simulink model "ClimateControlSystem_Standalone"  (R2026a)
settings: Solver=FixedStepAuto  StopTime=300  FixedStep=0.001  MaxStep=1e-4  RelTol=1e-4  AbsTol=1e-4  EnableMultiTasking=on
PreLoadFcn:
  | % NXP_MBDT_S32K3 callback: DO NOT REMOVE
  | mbd_s32k3.common.nxp.model_callbacks.preLoadFcn();
PostLoadFcn:
  | % NXP_MBDT_S32K3 callback: DO NOT REMOVE
  | mbd_s32k3.common.nxp.model_callbacks.postLoadFcn();
InitFcn:
  | % NXP_MBDT_S32K3 callback: DO NOT REMOVE
  | mbd_s32k3.common.nxp.model_callbacks.initFcn();
undefined symbols (not defined in the file or in its folder): DiscIntNeverNeededParam
libraries: mbd_s32k3_io_library x12, mbd_s32k3_isr_library x2, mbd_s32k3_utility_library x1
settings Model: DataDictionary=ClimateControlSystem_Standalone.sldd  PacingRate=1.100000  ExtModeTrigMode=oneshot  ExtModeArmWhenConnect=off  Creator=The MathWorks, Inc.  LastModifiedBy=nxa06644
settings SolverCC: MinimalZcImpactIntegration=on
settings DataIOCC: SignalLoggingName=sigsOut
settings OptimizationCC: InitFltsAndDblsToZero=on  EfficientMapNaN2IntZero=off
settings DebuggingCC: AlgebraicLoopMsg=error  SaveWithParameterizedLinksMsg=none  MultiTaskDSMMsg=warning  MultiTaskCondExecSysMsg=none  SubsystemReferenceDiagnosticForUnitTest=warning
settings HardwareCC: ProdLargestAtomicInteger=Long  ProdLargestAtomicFloat=Double  ProdHWDeviceType=ARM Compatible->ARM Cortex
settings RTWCC: SystemTargetFile=ert.tlc  HardwareBoard=NXP S32K3xx  TLCOptions=-aInlineSetEventsForThisBaseRateFcn=TLC_FALSE -aSuppressMultiTaskScheduler=TLC_FALSE -aRateBasedStepFcn=1  Toolchain=S32DS GCC  BuildConfiguration=Faster Runs  PortableWordSizes=on  Description=Embedded Coder
settings ERTTargetCC: ExtModeTransport=3.0  ERTSrcFileBannerTemplate=mbd_s32k3_ert_code_template.cgt  ERTHdrFileBannerTemplate=mbd_s32k3_ert_code_template.cgt  ERTDataSrcFileTemplate=mbd_s32k3_ert_code_template.cgt  ERTDataHdrFileTemplate=mbd_s32k3_ert_code_template.cgt  SupportContinuousTime=on
settings SimscapeCC: SimscapeNominalValues="[{\"value\":\"1\",\"unit\":\"A\"},{\"value\":\"1\",\"unit\":\"bar\"},{\"value\":\"1\",\"unit\":\"cm^2\"},{\"value\":\"1\",\"unit\":\"cm^3/s\"},{\"value\":\"1\",\"unit\":\"kJ/kg\"},{\"value\":\"1\",\"unit\":\"kW\"},{\"value\":\"1\",\"unit\":\"l\"},{\"value\":\"1\",\"unit\":\"N\"},{\"value\":\"1\",\"unit\":\"N*m\"},{\"value\":\"1\",\"unit\":\"V\"}]"  SimscapeLogName=simlog_sldemo_auto_climate_elec  SimscapeLogLimitData=off  SimscapeLogDataHistory=5000.0

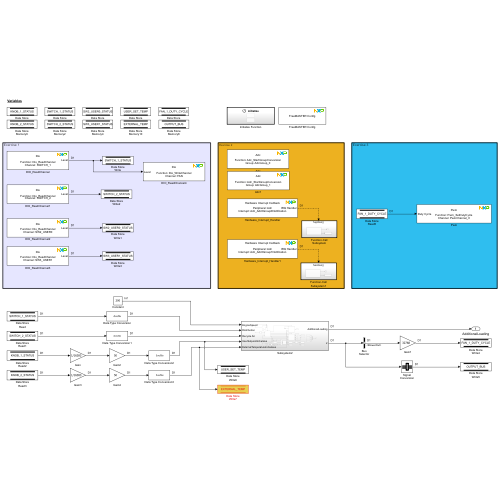
[thumbnail: Simulink's stored preview of the top-level diagram]
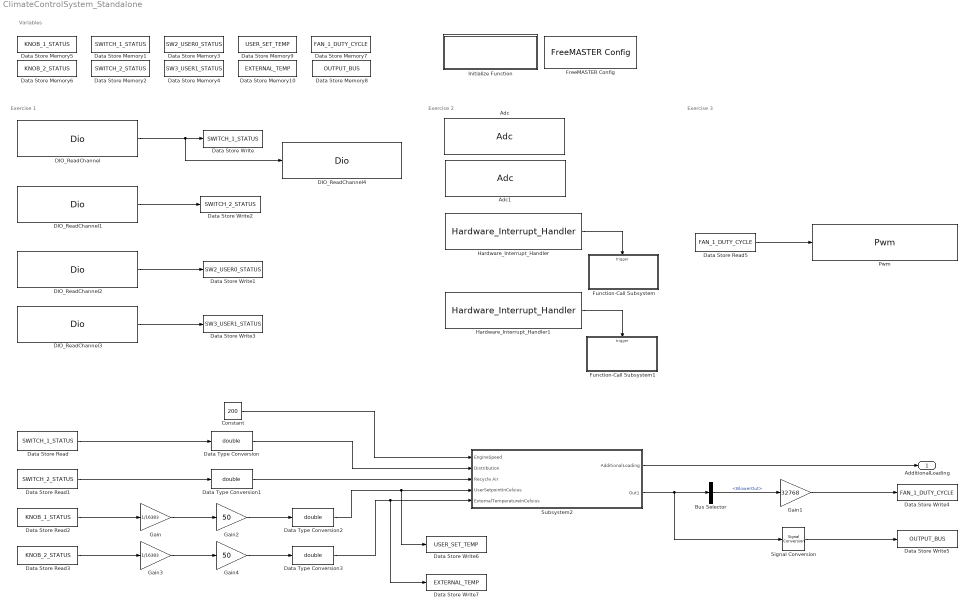
== system ClimateControlSystem_Standalone ==
  note: Exercise 2
  note: Variables
  note: Exercise 1
  note: Exercise 3
  Adc : mbd_s32k3_io_library/Adc  api_func=Adc_StartGroupConversion  hw_unit=AdcHwUnit_0  group=AdcGroup_0  channel=AdcChannel_KNOB_1  threshold_control=No ADC threshold control configured  power_state=ADC_FULL_POWER  ctu_unit=No CTU Unit configured  ctu_trigger=AdcHwTrigger_0  ctu_fifo_idx=No CTU FIFO available  text=<binary blob, 12330 chars, not shown>
      settings: SourceProductName=IO Blocks
  Adc1 : mbd_s32k3_io_library/Adc  api_func=Adc_StartGroupConversion  hw_unit=AdcHwUnit_0  group=AdcGroup_1  channel=AdcChannel_KNOB_1  threshold_control=No ADC threshold control configured  power_state=ADC_FULL_POWER  ctu_unit=No CTU Unit configured  ctu_trigger=AdcHwTrigger_0  ctu_fifo_idx=No CTU FIFO available  text=<binary blob, 12330 chars, not shown>
      settings: SourceProductName=IO Blocks
  Bus Selector : BusSelector  OutputSignals=BlowerOut
  Constant : Constant  Value=200
  DIO_ReadChannel : mbd_s32k3_io_library/Dio  Priority=0  api_func=Dio_ReadChannel  channel=SWITCH_1  channel_group=No channel groups configured  port=PTA_H  gpioSim=off  text=<binary blob, 2169 chars, not shown>
      settings: SourceProductName=IO Blocks
  DIO_ReadChannel1 : mbd_s32k3_io_library/Dio  Priority=0  api_func=Dio_ReadChannel  channel=SWITCH_2  channel_group=No channel groups configured  port=PTA_H  gpioSim=off  text=<binary blob, 2169 chars, not shown>
      settings: SourceProductName=IO Blocks
  DIO_ReadChannel2 : mbd_s32k3_io_library/Dio  Priority=0  api_func=Dio_ReadChannel  channel=SW2_USER0  channel_group=No channel groups configured  port=PTA_H  gpioSim=off  text=<binary blob, 2169 chars, not shown>
      settings: SourceProductName=IO Blocks
  DIO_ReadChannel3 : mbd_s32k3_io_library/Dio  Priority=0  api_func=Dio_ReadChannel  channel=SW3_USER1  channel_group=No channel groups configured  port=PTA_H  gpioSim=off  text=<binary blob, 2169 chars, not shown>
      settings: SourceProductName=IO Blocks
  DIO_ReadChannel4 : mbd_s32k3_io_library/Dio  Priority=0  api_func=Dio_WriteChannel  channel=FAN  channel_group=No channel groups configured  port=PTA_H  gpioSim=off  text=<binary blob, 2169 chars, not shown>
      settings: SourceProductName=IO Blocks
  Data Store Memory1 : DataStoreMemory  DataStoreName=SWITCH_1_STATUS  ReadBeforeWriteMsg=warning  WriteAfterWriteMsg=warning  WriteAfterReadMsg=warning  ShowAdditionalParam=off  OutDataTypeStr=uint8
  Data Store Memory10 : DataStoreMemory  DataStoreName=EXTERNAL_TEMP  ReadBeforeWriteMsg=warning  WriteAfterWriteMsg=warning  WriteAfterReadMsg=warning  ShowAdditionalParam=off  OutDataTypeStr=double
  Data Store Memory2 : DataStoreMemory  DataStoreName=SWITCH_2_STATUS  ReadBeforeWriteMsg=warning  WriteAfterWriteMsg=warning  WriteAfterReadMsg=warning  ShowAdditionalParam=off  OutDataTypeStr=uint8
  Data Store Memory3 : DataStoreMemory  DataStoreName=SW2_USER0_STATUS  ReadBeforeWriteMsg=warning  WriteAfterWriteMsg=warning  WriteAfterReadMsg=warning  ShowAdditionalParam=off  OutDataTypeStr=uint8
  Data Store Memory4 : DataStoreMemory  DataStoreName=SW3_USER1_STATUS  ReadBeforeWriteMsg=warning  WriteAfterWriteMsg=warning  WriteAfterReadMsg=warning  ShowAdditionalParam=off  OutDataTypeStr=uint8
  Data Store Memory5 : DataStoreMemory  DataStoreName=KNOB_1_STATUS  ReadBeforeWriteMsg=warning  WriteAfterWriteMsg=warning  WriteAfterReadMsg=warning  ShowAdditionalParam=off  OutDataTypeStr=uint16
  Data Store Memory6 : DataStoreMemory  DataStoreName=KNOB_2_STATUS  ReadBeforeWriteMsg=warning  WriteAfterWriteMsg=warning  WriteAfterReadMsg=warning  ShowAdditionalParam=off  OutDataTypeStr=uint16
  Data Store Memory7 : DataStoreMemory  DataStoreName=FAN_1_DUTY_CYCLE  ReadBeforeWriteMsg=warning  WriteAfterWriteMsg=warning  WriteAfterReadMsg=warning  ShowAdditionalParam=off  OutDataTypeStr=uint16
  Data Store Memory8 : DataStoreMemory  DataStoreName=OUTPUT_BUS  ReadBeforeWriteMsg=warning  WriteAfterWriteMsg=warning  WriteAfterReadMsg=warning  ShowAdditionalParam=off  OutDataTypeStr=Bus: OutputBus
  Data Store Memory9 : DataStoreMemory  DataStoreName=USER_SET_TEMP  ReadBeforeWriteMsg=warning  WriteAfterWriteMsg=warning  WriteAfterReadMsg=warning  ShowAdditionalParam=off  OutDataTypeStr=double
  Data Store Read : DataStoreRead  DataStoreName=SWITCH_1_STATUS  IndexOptions=Index vector (dialog)  Indices=1  OutputSizes=1
  Data Store Read1 : DataStoreRead  DataStoreName=SWITCH_2_STATUS  IndexOptions=Index vector (dialog)  Indices=1  OutputSizes=1
  Data Store Read2 : DataStoreRead  DataStoreName=KNOB_1_STATUS  IndexOptions=Index vector (dialog)  Indices=1  OutputSizes=1
  Data Store Read3 : DataStoreRead  DataStoreName=KNOB_2_STATUS  IndexOptions=Index vector (dialog)  Indices=1  OutputSizes=1
  Data Store Read5 : DataStoreRead  DataStoreName=FAN_1_DUTY_CYCLE  IndexOptions=Index vector (dialog)  Indices=1  OutputSizes=1
  Data Store Write : DataStoreWrite  DataStoreName=SWITCH_1_STATUS  IndexOptions=Index vector (dialog)  Indices=1  OutputSizes=1
  Data Store Write1 : DataStoreWrite  DataStoreName=SW2_USER0_STATUS  IndexOptions=Index vector (dialog)  Indices=1  OutputSizes=1
  Data Store Write2 : DataStoreWrite  DataStoreName=SWITCH_2_STATUS  IndexOptions=Index vector (dialog)  Indices=1  OutputSizes=1
  Data Store Write3 : DataStoreWrite  DataStoreName=SW3_USER1_STATUS  IndexOptions=Index vector (dialog)  Indices=1  OutputSizes=1
  Data Store Write4 : DataStoreWrite  DataStoreName=FAN_1_DUTY_CYCLE  IndexOptions=Index vector (dialog)  Indices=1  OutputSizes=1
  Data Store Write5 : DataStoreWrite  DataStoreName=OUTPUT_BUS  IndexOptions=Index vector (dialog)  Indices=1  OutputSizes=1
  Data Store Write6 : DataStoreWrite  DataStoreName=USER_SET_TEMP  IndexOptions=Index vector (dialog)  Indices=1  OutputSizes=1
  Data Store Write7 : DataStoreWrite  DataStoreName=EXTERNAL_TEMP  IndexOptions=Index vector (dialog)  Indices=1  OutputSizes=1
  Data Type Conversion{,1..3} (4 alike) : DataTypeConversion  OutDataTypeStr=double  SaturateOnIntegerOverflow=off  RndMeth=Floor
  FreeMASTER Config : mbd_s32k3_utility_library/FreeMASTER blocks/FreeMASTER Config  connection_type=Serial  instance=LPUART_6  baudrate=115200  isr_prio=5  cantxid=0x7aa  cantxidext=on  cantxobj=5  canrxid=0x7aa  canrxidext=on  canrxobj=5  mode=Short Interrupt  scope_use=1  scope_max_vars=8  automatic_buff_size=on  buff_size=255  default_rfifo_size=on  rfifo_size=32
      settings: SourceProductName=Utility Blocks
  Function-Call Subsystem : Subsystem  TreatAsAtomicUnit=on
  Function-Call Subsystem1 : Subsystem  TreatAsAtomicUnit=on
  Gain : Gain  Gain=1/16383  OutDataTypeStr=single
  Gain1 : Gain  Gain=32768  OutDataTypeStr=uint16
  Gain2 : Gain  Gain=50  OutDataTypeStr=double
  Gain3 : Gain  Gain=1/16383  OutDataTypeStr=single
  Gain4 : Gain  Gain=50  OutDataTypeStr=double
  Hardware_Interrupt_Handler : mbd_s32k3_isr_library/Hardware_Interrupt_Handler  blockCbk=0  irqGroup=Adc  irqHandlers=Adc_Adc0Group0Notification  irqSim=off  text=<binary blob, 12330 chars, not shown>
      settings: SourceProductName=ISR Blocks
  Hardware_Interrupt_Handler1 : mbd_s32k3_isr_library/Hardware_Interrupt_Handler  blockCbk=0  irqGroup=Adc  irqHandlers=Adc_Adc0Group1Notification  irqSim=off  text=<binary blob, 12330 chars, not shown>
      settings: SourceProductName=ISR Blocks
  Initialize Function : Subsystem  TreatAsAtomicUnit=on
  Pwm : mbd_s32k3_io_library/Pwm  api_func=Pwm_SetDutyCycle  channel=PwmChannel_0  notification=PWM_RISING_EDGE  moduleId=PWM_EMIOS_INSTANCE_0  prescalerType=PWM_PRIMARY_PRESCALER  fault=PWM_FLEXPWM_0_FAULT_INPUT_0  text=<binary blob, 3846 chars, not shown>
      settings: SourceProductName=IO Blocks
  Signal Conversion : SignalConversion  ConversionOutput=Nonvirtual bus  OutDataTypeStr=Bus: OutputBus  OverrideOpt=off
  Subsystem2 : Subsystem
  AdditionalLoading : Outport  OutDataTypeStr=double  PortDimensions=1  VectorParamsAs1DForOutWhenUnconnected=off
  wires:
  Constant/1 -> Subsystem2/1(EngineSpeed)
  Data Store Read/1 -> Data Type Conversion/1
  Data Store Read1/1 -> Data Type Conversion1/1
  Data Store Read2/1 -> Gain/1
  Data Store Read3/1 -> Gain3/1
  Subsystem2/1(AdditionalLoading) -> AdditionalLoading/1
  Subsystem2/2(Out1) -> Signal Conversion/1, Bus Selector/1
  Hardware_Interrupt_Handler1/1 -> Function-Call Subsystem1/Trigger
  DIO_ReadChannel/1 -> DIO_ReadChannel4/1, Data Store Write/1
  DIO_ReadChannel1/1 -> Data Store Write2/1
  Hardware_Interrupt_Handler/1 -> Function-Call Subsystem/Trigger
  DIO_ReadChannel2/1 -> Data Store Write1/1
  DIO_ReadChannel3/1 -> Data Store Write3/1
  Data Store Read5/1 -> Pwm/1
  Bus Selector/1 -> Gain1/1  "<BlowerOut>"
  Gain1/1 -> Data Store Write4/1
  Gain/1 -> Gain2/1
  Gain2/1 -> Data Type Conversion2/1
  Gain3/1 -> Gain4/1
  Gain4/1 -> Data Type Conversion3/1
  Data Type Conversion/1 -> Subsystem2/2(Distribution)
  Data Type Conversion1/1 -> Subsystem2/3(Recycle Air)
  Data Type Conversion2/1 -> Subsystem2/4(UserSetpointInCelsius), Data Store Write6/1
  Data Type Conversion3/1 -> Data Store Write7/1, Subsystem2/5(ExternalTemperatureInCelsius)
  Signal Conversion/1 -> Data Store Write5/1

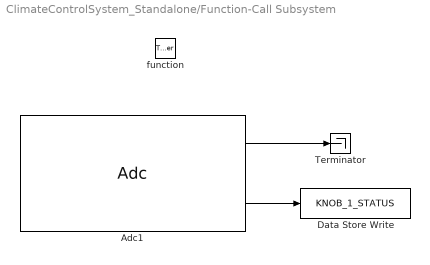
== system ClimateControlSystem_Standalone/Function-Call Subsystem ==
  function : TriggerPort  TriggerType=function-call  VariantControl=(inherit)
  Adc1 : mbd_s32k3_io_library/Adc  api_func=Adc_ReadGroup  hw_unit=AdcHwUnit_0  group=AdcGroup_0  channel=AdcChannel_KNOB_1  threshold_control=No ADC threshold control configured  power_state=ADC_FULL_POWER  ctu_unit=No CTU Unit configured  ctu_trigger=AdcHwTrigger_0  ctu_fifo_idx=No CTU FIFO available  text=<binary blob, 12330 chars, not shown>
      settings: SourceProductName=IO Blocks
  Data Store Write : DataStoreWrite  DataStoreName=KNOB_1_STATUS  IndexOptions=Index vector (dialog)  Indices=1  OutputSizes=1
  Terminator : Terminator
  wires:
  Adc1/2 -> Data Store Write/1
  Adc1/1 -> Terminator/1

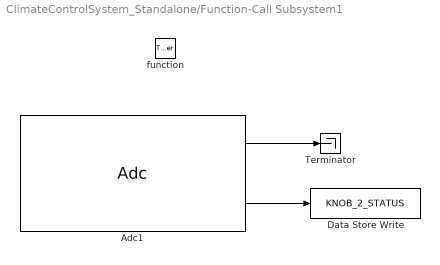
== system ClimateControlSystem_Standalone/Function-Call Subsystem1 ==
  function : TriggerPort  TriggerType=function-call  VariantControl=(inherit)
  Adc1 : mbd_s32k3_io_library/Adc  api_func=Adc_ReadGroup  hw_unit=AdcHwUnit_0  group=AdcGroup_1  channel=AdcChannel_KNOB_1  threshold_control=No ADC threshold control configured  power_state=ADC_FULL_POWER  ctu_unit=No CTU Unit configured  ctu_trigger=AdcHwTrigger_0  ctu_fifo_idx=No CTU FIFO available  text=<binary blob, 12330 chars, not shown>
      settings: SourceProductName=IO Blocks
  Data Store Write : DataStoreWrite  DataStoreName=KNOB_2_STATUS  IndexOptions=Index vector (dialog)  Indices=1  OutputSizes=1
  Terminator : Terminator
  wires:
  Adc1/2 -> Data Store Write/1
  Adc1/1 -> Terminator/1

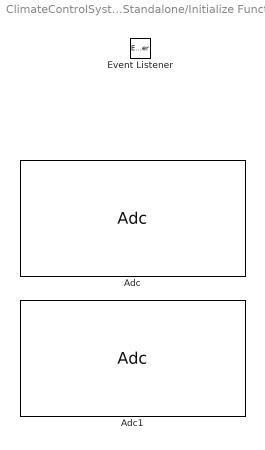
== system ClimateControlSystem_Standalone/Initialize Function ==
  Adc : mbd_s32k3_io_library/Adc  api_func=Adc_EnableGroupNotification  hw_unit=AdcHwUnit_0  group=AdcGroup_0  channel=AdcChannel_KNOB_1  threshold_control=No ADC threshold control configured  power_state=ADC_FULL_POWER  ctu_unit=No CTU Unit configured  ctu_trigger=AdcHwTrigger_0  ctu_fifo_idx=No CTU FIFO available  text=<binary blob, 12330 chars, not shown>
      settings: SourceProductName=IO Blocks
  Adc1 : mbd_s32k3_io_library/Adc  api_func=Adc_EnableGroupNotification  hw_unit=AdcHwUnit_0  group=AdcGroup_1  channel=AdcChannel_KNOB_1  threshold_control=No ADC threshold control configured  power_state=ADC_FULL_POWER  ctu_unit=No CTU Unit configured  ctu_trigger=AdcHwTrigger_0  ctu_fifo_idx=No CTU FIFO available  text=<binary blob, 12330 chars, not shown>
      settings: SourceProductName=IO Blocks
  Event Listener : EventListener  DisableCoverage=on  EventName=reset

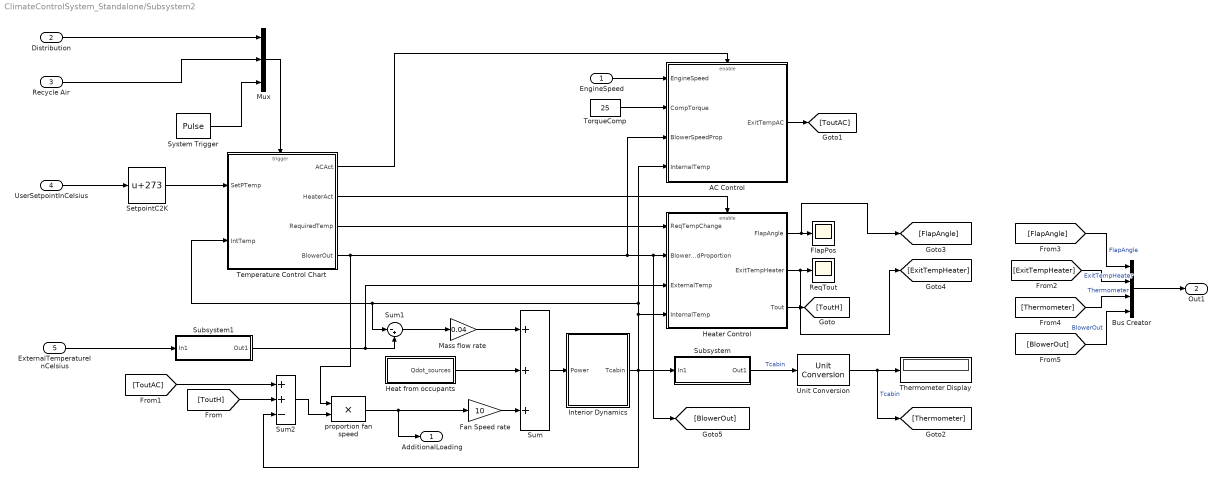
== system ClimateControlSystem_Standalone/Subsystem2 ==
  EngineSpeed : Inport  OutDataTypeStr=double  PortDimensions=1
  Distribution : Inport  Port=2  OutDataTypeStr=double
  Recycle Air : Inport  Port=3  OutDataTypeStr=double
  UserSetpointInCelsius : Inport  Port=4
  ExternalTemperatureInCelsius : Inport  Port=5
  AC Control : Subsystem  TreatAsAtomicUnit=on
  Bus Creator : BusCreator  Inputs=4  OutDataTypeStr=Bus: OutputBus
  Fan Speed rate : Gain  Gain=10  SaturateOnIntegerOverflow=on  OutDataTypeStr=Inherit: Same as input  ParamDataTypeStr=Inherit: Same as input
  FlapPos : Scope
      settings: ActiveDisplayYMinimum=-1  ActiveDisplayYMaximum=1
  Heat from occupants : Subsystem  mask(Heat from occupants){N=1}
      mask prompts: N "Number of occupants:"
      settings: AttributesFormatString=No. of occupants: %<N>
      mask Display: disp('Heat Sources')
  Heater Control : Subsystem  TreatAsAtomicUnit=on
  Interior Dynamics : Subsystem  mask(Vehicle Cabin Dynamics){}
      mask Display: image('$imagefile') % use "Edit Image" on toolstrip to change
  Mass flow rate : Gain  Gain=0.04  SaturateOnIntegerOverflow=on  OutDataTypeStr=Inherit: Same as input  ParamDataTypeStr=Inherit: Same as input
  Mux : Mux  Inputs=3
  ReqTout : Scope
      settings: ActiveDisplayYMinimum=-1  ActiveDisplayYMaximum=1
  SetpointC2K : Bias  Bias=273  SaturateOnIntegerOverflow=off
  Subsystem : Subsystem
      mask Display: disp('Kelvin to Celsius')
  Subsystem1 : Subsystem
      mask Display: disp('Celsius to Kelvin')
  Sum : Sum  Inputs=+++  InputSameDT=on  SaturateOnIntegerOverflow=on  OutDataTypeStr=Inherit: Same as first input
  Sum1 : Sum  Inputs=|-+  InputSameDT=on  SaturateOnIntegerOverflow=on  OutDataTypeStr=Inherit: Same as first input
  Sum2 : Sum  Inputs=++-  InputSameDT=on  SaturateOnIntegerOverflow=on  OutDataTypeStr=Inherit: Same as first input
  System Trigger : DiscretePulseGenerator  SampleTime=-1
  Temperature Control Chart : Stateflow chart  TreatAsAtomicUnit=on
  Thermometer Display : Display
  TorqueComp : Constant  Value=25
  Unit Conversion : UnitConversion
  proportion fan speed : Product  InputSameDT=on  SaturateOnIntegerOverflow=on  OutDataTypeStr=Inherit: Same as first input
  AdditionalLoading : Outport  OutDataTypeStr=double  PortDimensions=1  VectorParamsAs1DForOutWhenUnconnected=off
  Out1 : Outport  Port=2  OutDataTypeStr=Bus: OutputBus
  wires:
  AC Control/1(ExitTempAC) -> [ToutAC]
  [BlowerOut] -> Bus Creator/4  "BlowerOut"
  Interior Dynamics/1("Tcabin ") -> Heater Control/4(InternalTemp), Temperature Control Chart/2(IntTemp), Sum1/1, AC Control/4(InternalTemp), Sum2/3, Subsystem/1(In1)
  TorqueComp/1 -> AC Control/2(CompTorque)
  proportion fan speed/1 -> AdditionalLoading/1, Fan Speed rate/1
  Heater Control/2(ExitTempHeater) -> [ExitTempHeater], ReqTout/1
  [Thermometer] -> Bus Creator/3  "Thermometer"
  EngineSpeed/1 -> AC Control/1(EngineSpeed)
  Heater Control/3(Tout) -> [ToutH]
  Fan Speed rate/1 -> Sum/3
  Sum/1 -> Interior Dynamics/1(Power)
  Recycle Air/1 -> Mux/2
  Sum1/1 -> Mass flow rate/1
  Subsystem/1(Out1) -> Unit Conversion/1  "Tcabin"
  SetpointC2K/1 -> Temperature Control Chart/1(SetPTemp)
  Heater Control/1(FlapAngle) -> [FlapAngle], FlapPos/1
  Sum2/1 -> proportion fan speed/2
  Unit Conversion/1 -> [Thermometer], Thermometer Display/1  "Tcabin"
  Temperature Control Chart/3(RequiredTemp) -> Heater Control/1(ReqTempChange)
  [ToutH] -> Sum2/2
  Subsystem1/1(Out1) -> Heater Control/3(ExternalTemp), Sum1/2
  [ExitTempHeater] -> Bus Creator/2  "ExitTempHeater"
  Distribution/1 -> Mux/1
  Bus Creator/1 -> Out1/1
  Temperature Control Chart/4(BlowerOut) -> [BlowerOut], Heater Control/2(BlowerSpeedProportion), AC Control/3(BlowerSpeedProp), proportion fan speed/1
  ExternalTemperatureInCelsius/1 -> Subsystem1/1(In1)
  Temperature Control Chart/1(" ACAct") -> AC Control/Enable
  Mass flow rate/1 -> Sum/1
  Mux/1 -> Temperature Control Chart/Trigger
  UserSetpointInCelsius/1 -> SetpointC2K/1
  Heat from occupants/1(Qdot_sources) -> Sum/2
  [ToutAC] -> Sum2/1
  System Trigger/1 -> Mux/3
  [FlapAngle] -> Bus Creator/1  "FlapAngle"
  Temperature Control Chart/2(" HeaterAct") -> Heater Control/Enable

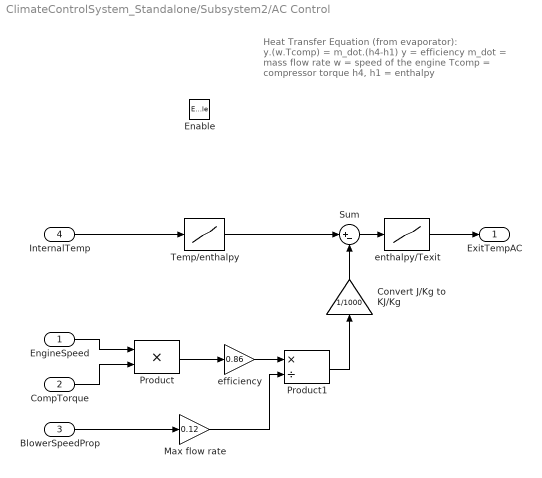
== system ClimateControlSystem_Standalone/Subsystem2/AC Control ==
  note: Heat Transfer Equation (from evaporator):
      |
      | y.(w.Tcomp) = m_dot.(h4-h1)
      |
      | y = efficiency
      | m_dot = mass flow rate
      | w = speed of the engine
      | Tcomp = compressor torque
      | h4, h1 = enthalpy
  EngineSpeed : Inport
  CompTorque : Inport  Port=2
  BlowerSpeedProp : Inport  Port=3
  InternalTemp : Inport  Port=4
  Enable : EnablePort  StatesWhenEnabling=reset  PropagateVarSize=During execution  ZeroCross=off
  Convert J/Kg to KJ/Kg : Gain  Gain=1/1000
  Max flow rate : Gain  Gain=0.12  SaturateOnIntegerOverflow=on  OutDataTypeStr=Inherit: Same as input  ParamDataTypeStr=Inherit: Same as input
  Product : Product  InputSameDT=on  SaturateOnIntegerOverflow=on  OutDataTypeStr=Inherit: Same as first input
  Product1 : Product  Inputs=*/  InputSameDT=on  SaturateOnIntegerOverflow=on  OutDataTypeStr=Inherit: Same as first input
  Sum : Sum  Inputs=|+-  InputSameDT=on  SaturateOnIntegerOverflow=on  OutDataTypeStr=Inherit: Same as first input
  Temp/enthalpy : Lookup_n-D  NumberOfTableDimensions=1  BreakpointsForDimension1=[220 230 240 250 260 270 280 285 290 295 300 305 310 315 320]  Table=[219.97 230.02 240.02 250.05 260.09 270.11 280.13 285.14 290.16 295.17 300.19 305.22 310.24 315.27 320.29]  SaturateOnIntegerOverflow=on
  efficiency : Gain  Gain=0.86  SaturateOnIntegerOverflow=on  OutDataTypeStr=Inherit: Same as input  ParamDataTypeStr=Inherit: Same as input
  enthalpy/Texit : Lookup_n-D  NumberOfTableDimensions=1  BreakpointsForDimension1=[219.97 230.02 240.02 250.05 260.09 270.11 280.13 285.14 290.16 295.17 300.19 305.22 310.24 315.27 320.29]  Table=[220 230 240 250 260 270 280 285 290 295 300 305 310 315 320]  SaturateOnIntegerOverflow=on
  ExitTempAC : Outport  OutputWhenDisabled=reset  InitialOutput=0  VectorParamsAs1DForOutWhenUnconnected=off
  wires:
  Convert J/Kg to KJ/Kg/1 -> Sum/2
  Sum/1 -> enthalpy/Texit/1
  Product1/1 -> Convert J/Kg to KJ/Kg/1
  Temp/enthalpy/1 -> Sum/1
  InternalTemp/1 -> Temp/enthalpy/1
  enthalpy/Texit/1 -> ExitTempAC/1
  Max flow rate/1 -> Product1/2
  BlowerSpeedProp/1 -> Max flow rate/1
  efficiency/1 -> Product1/1
  Product/1 -> efficiency/1
  CompTorque/1 -> Product/2
  EngineSpeed/1 -> Product/1

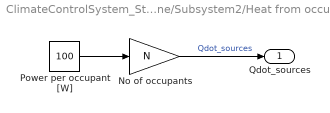
== system ClimateControlSystem_Standalone/Subsystem2/Heat from occupants ==
  No of occupants : Gain  Gain=N  SaturateOnIntegerOverflow=on  OutDataTypeStr=Inherit: Same as input  ParamDataTypeStr=Inherit: Same as input
  Power per occupant [W] : Constant  Value=100
  Qdot_sources : Outport  VectorParamsAs1DForOutWhenUnconnected=off
  wires:
  Power per occupant [W]/1 -> No of occupants/1
  No of occupants/1 -> Qdot_sources/1  "Qdot_sources"

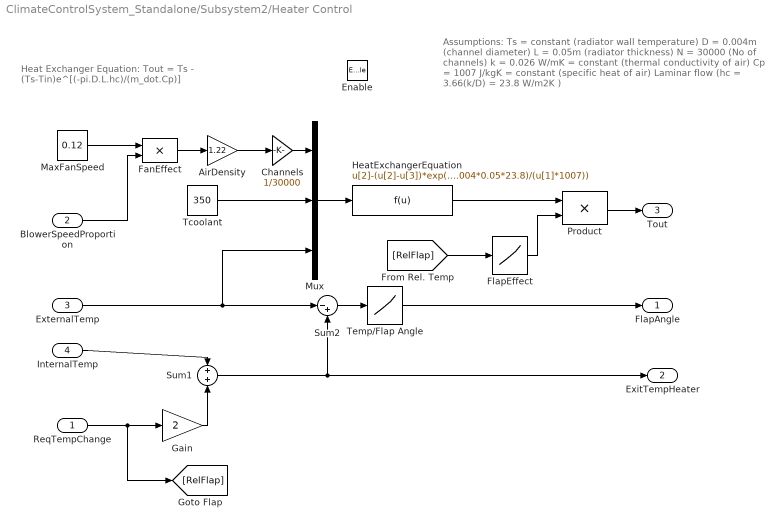
== system ClimateControlSystem_Standalone/Subsystem2/Heater Control ==
  note: Assumptions:
      | Ts = constant (radiator wall temperature)
      | D = 0.004m (channel diameter)
      | L = 0.05m (radiator thickness)
      | N = 30000 (No of channels)
      |
      | k = 0.026 W/mK = constant (thermal conductivity of air)
      | Cp = 1007 J/kgK = constant (specific heat of air)
      | Laminar flow (hc = 3.66(k/D) = 23.8 W/m2K )
  note: Heat Exchanger Equation:
      | Tout = Ts - (Ts-Tin)e^[(-pi.D.L.hc)/(m_dot.Cp)]
  ReqTempChange : Inport
  BlowerSpeedProportion : Inport  Port=2
  ExternalTemp : Inport  Port=3
  InternalTemp : Inport  Port=4
  Enable : EnablePort  StatesWhenEnabling=reset  PropagateVarSize=During execution  ZeroCross=off
  AirDensity : Gain  Gain=1.22  SaturateOnIntegerOverflow=on  OutDataTypeStr=Inherit: Same as input  ParamDataTypeStr=Inherit: Same as input
  Channels : Gain  Gain=1/30000  SaturateOnIntegerOverflow=on  OutDataTypeStr=Inherit: Same as input  ParamDataTypeStr=Inherit: Same as input
  FanEffect : Product  InputSameDT=on  SaturateOnIntegerOverflow=on  OutDataTypeStr=Inherit: Same as first input
  FlapEffect : Lookup_n-D  NumberOfTableDimensions=1  BreakpointsForDimension1="[0 3 5 10 50  90 100 200 ]"  Table="[0 300 100  10 10  10 3 1]"  SaturateOnIntegerOverflow=on
  Gain : Gain  Gain=2  SaturateOnIntegerOverflow=on  OutDataTypeStr=Inherit: Same as input  ParamDataTypeStr=Inherit: Same as input
  HeatExchangerEquation : Fcn  Expr=u[2]-(u[2]-u[3])*exp(-(pi*0.004*0.05*23.8)/(u[1]*1007))
  MaxFanSpeed : Constant  Value=0.12
  Mux : Mux  Inputs=3
  Product : Product  InputSameDT=on  SaturateOnIntegerOverflow=on  OutDataTypeStr=Inherit: Same as first input
  Sum1 : Sum  InputSameDT=on  SaturateOnIntegerOverflow=on  OutDataTypeStr=Inherit: Same as first input
  Sum2 : Sum  Inputs=|-+  InputSameDT=on  SaturateOnIntegerOverflow=on  OutDataTypeStr=Inherit: Same as first input
  "Tcoolant " : Constant  Value=350
  Temp/Flap Angle : Lookup_n-D  NumberOfTableDimensions=1  BreakpointsForDimension1=[0 10 20 30 40 50 60 75 100 200]  Table=[0 20 30 45 60 75 90 90 90 90]  SaturateOnIntegerOverflow=on
  FlapAngle : Outport  OutputWhenDisabled=reset  InitialOutput=0  VectorParamsAs1DForOutWhenUnconnected=off
  ExitTempHeater : Outport  Port=2  OutputWhenDisabled=reset  InitialOutput=0  VectorParamsAs1DForOutWhenUnconnected=off
  Tout : Outport  Port=3  OutputWhenDisabled=reset  InitialOutput=0  VectorParamsAs1DForOutWhenUnconnected=off
  wires:
  HeatExchangerEquation/1 -> Product/1
  ExternalTemp/1 -> Mux/3, Sum2/1
  BlowerSpeedProportion/1 -> FanEffect/2
  MaxFanSpeed/1 -> FanEffect/1
  FanEffect/1 -> AirDensity/1
  Mux/1 -> HeatExchangerEquation/1
  AirDensity/1 -> Channels/1
  Channels/1 -> Mux/1
  "Tcoolant "/1 -> Mux/2
  Product/1 -> Tout/1
  Temp/Flap Angle/1 -> FlapAngle/1
  Sum2/1 -> Temp/Flap Angle/1
  InternalTemp/1 -> Sum1/1
  Gain/1 -> Sum1/2
  Sum1/1 -> ExitTempHeater/1, Sum2/2
  ReqTempChange/1 -> Gain/1, [RelFlap]
  FlapEffect/1 -> Product/2
  [RelFlap] -> FlapEffect/1

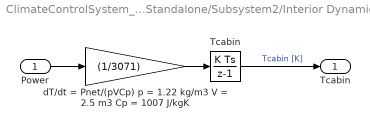
== system ClimateControlSystem_Standalone/Subsystem2/Interior Dynamics ==
  Power : Inport
  Tcabin : DiscreteIntegrator  InitialCondition=273+29  SampleTime=-1  ICPrevOutput=DiscIntNeverNeededParam  ICPrevScaledInput=DiscIntNeverNeededParam
  dT/dt = Pnet/(pVCp) p = 1.22 kg/m3 V = 2.5 m3 Cp = 1007 J/kgK : Gain  Gain=(1/3071)  SaturateOnIntegerOverflow=on  OutDataTypeStr=Inherit: Same as input  ParamDataTypeStr=Inherit: Same as input
  "Tcabin " : Outport  VectorParamsAs1DForOutWhenUnconnected=off
  wires:
  Power/1 -> dT/dt = Pnet/(pVCp) p = 1.22 kg/m3 V = 2.5 m3 Cp = 1007 J/kgK/1
  dT/dt = Pnet/(pVCp) p = 1.22 kg/m3 V = 2.5 m3 Cp = 1007 J/kgK/1 -> Tcabin/1
  Tcabin/1 -> "Tcabin "/1  "Tcabin [K]"

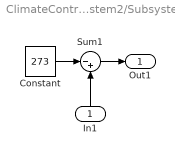
== system ClimateControlSystem_Standalone/Subsystem2/Subsystem ==
  In1 : Inport
  Constant : Constant  Value=273
  Sum1 : Sum  Inputs=|-+  InputSameDT=on  SaturateOnIntegerOverflow=on  OutDataTypeStr=Inherit: Same as first input
  Out1 : Outport  VectorParamsAs1DForOutWhenUnconnected=off
  wires:
  Sum1/1 -> Out1/1
  In1/1 -> Sum1/2
  Constant/1 -> Sum1/1

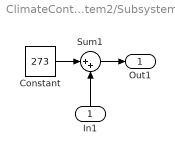
== system ClimateControlSystem_Standalone/Subsystem2/Subsystem1 ==
  In1 : Inport
  Constant : Constant  Value=273
  Sum1 : Sum  Inputs=|++  InputSameDT=on  SaturateOnIntegerOverflow=on  OutDataTypeStr=Inherit: Same as first input
  Out1 : Outport  VectorParamsAs1DForOutWhenUnconnected=off
  wires:
  Constant/1 -> Sum1/1
  In1/1 -> Sum1/2
  Sum1/1 -> Out1/1

== stateflow chart ClimateControlSystem_Standalone/Subsystem2/Temperature Control Chart ==
  state Blower [parallel]
    during:setpoint_calc();
    settings: executionOrder=1
    state Blower_off
      entry:BlowerOut=0.0;
    state Blower_on
      state Blower_1
        entry:BlowerOut=0.2;
      state Blower_2
        entry:BlowerOut=0.4;
      state Blower_3
        entry:BlowerOut=0.6;
      state Blower_4
        entry:BlowerOut=0.8;
      state Blower_5
        entry:BlowerOut=1.0;
      (default) -> Blower_1
      Blower_on -> Blower_1 [order 5] : E[~in(Blower_1) && in_temp_range(1.5,5)]
      Blower_on -> Blower_2 [order 4] : E[~in(Blower_2) && in_temp_range(7,10)]
      Blower_on -> Blower_3 [order 3] : E[~in(Blower_3) && in_temp_range(12,15)]
      Blower_on -> Blower_4 [order 2] : E[~in(Blower_4) && in_temp_range(17,20)]
      Blower_on -> Blower_5 [order 1] : E[~in(Blower_5) && in_temp_range(22,200)]
    state setpoint_calc() [function]
      (default) -> (junction 51) : {RequiredTemp = SetPTemp-IntTemp;}
      (junction 51) -> (junction 48) [order 1] : [RequiredTemp<0.0]
          | {absTempDiff = -RequiredTemp;}
      (junction 51) -> (junction 49) [order 2] : {absTempDiff = RequiredTemp;}
    state b = in_temp_range(minTemp,maxTemp) [function]
      (default) -> (junction 50) : {b = (absTempDiff>minTemp) &&  ...
          |         (absTempDiff<maxTemp);}
    (default) -> Blower_off
    Blower_off -> Blower_on : E[absTempDiff<203 || absTempDiff>1]
    Blower_on -> Blower_off [order 1] : E[absTempDiff>203 || absTempDiff<=eps]
  state Heater_AC [parallel]
    settings: executionOrder=2
    state H_offAC_off
    state ACAct
    state HeaterAct
    ACAct -> H_offAC_off : E[SetPTemp-IntTemp>=-0.5]
    HeaterAct -> H_offAC_off : E[SetPTemp-IntTemp<=0.5]
    H_offAC_off -> HeaterAct [order 2] : E[SetPTemp-IntTemp>0.55]
    H_offAC_off -> ACAct [order 1] : E[SetPTemp-IntTemp<-0.55]
    (default) -> H_offAC_off
  state AirDist [parallel]
    settings: executionOrder=3
    state Feet
    state Face
    state Defrost
    (default) -> Face
    Feet -> Defrost : DistReq
    Face -> Feet : DistReq
    Defrost -> Face : DistReq
  state Recyc_Air [parallel]
    settings: executionOrder=4
    state Recyc_on
    state Recyc_off
    (default) -> Recyc_on
    Recyc_on -> Recyc_off [order 2] : RecycReq
    Recyc_off -> Recyc_on : RecycReq
    Recyc_on -> Recyc_off [order 1] : en(AirDist.Defrost)
  data: minTemp function_input double; b function_output boolean; maxTemp function_input double; ACAct output boolean; SetPTemp input double; IntTemp input double; HeaterAct output boolean; RequiredTemp output double; BlowerOut output double; absTempDiff local double
  events: DistReq input EITHER_EDGE_EVENT; RecycReq input EITHER_EDGE_EVENT; E input EITHER_EDGE_EVENT
